simulink library "ars"  (Simulink 8.1)
settings: Solver=ode1  StartTime=0.0  StopTime=Inf  FixedStep=0.001  RelTol=1e-3
PostLoadFcn:
  | , if any(exist('dsrtsu_mdlpostloadfcn', 'file') == [2, 3, 6]), try dsrtsu_mdlpostloadfcn('Execute', bdroot); catch fprintf('Error in PostLoadFcn (dsrtsu_mdlpostloadfcn) for model "%s":\n %s\n', bdroot, lasterr); end, end,
undefined symbols (not defined in the file or in its folder): KACC_RawFMLowerLimit_mps, KACC_RawFMUpperLimit_mps
libraries: hcu_lib x2, ssc x1, ddc x1, dch x1, rsd x1, rsa x1, rst x1
settings Model: DSRTSU_INTERNAL_RTI_VER=450  DSRTSU_INTERNAL_RTI_TYPE=rti1401  RTICANMMDATA=struct('GeneralSetupData',struct('modelroot','D:\ELN150201_TAIWAN\trunk\AdasDragon\software\sw_development\arch\app\acc','generalsettings',struct('filesettings',struct('destfolder',struct('Name','RTICANMM_FILES','Check',1),'buildfolder',struct('Name','.','Check',1),'AbsDestfolder',struct('Name','D:\ELN150201_TAIWAN\trunk\AdasDragon\software\sw_development\arch\app\acc\RTICANMM_FILES'),'AbsBuildfolder',struct('Name','D:\ELN150201_TAIWAN\trunk\AdasDragon\software\sw_development\arch\app\acc'))),'options',struct('addpaths',1,'rmpaths',1,'addtrcexclusion',logical(1),'cannavigator',struct('checkmonitoring',0),'show_usrtrc',0,'use_usrtrc',0),'advanced',struct('options',[1 1 1 1 1 1 1 1 1 1 1 1 1 1 1 1 1 1 1 1 1 1 1 1 1 1 1 1 1 1 1 1 1 1 1 1 1 1 1 1 1 1 1 1 1 1 1 1 1 1 1 1 1 1 1 1 1 1 1 1 1 1 1 1 1 1 1 1 1 1 1 1 1 1 1 1 1 1 1 1 1 1 1 1 1 1 1 1 1 1 1 1 1 1 1 1 1 1 1 1]),'MPSetup',{{}},'modelname','ars','block','ars'))  DSRTSU_INTERNAL_RTIFPGA=40  Creator=tescamilla  LastModifiedBy=AT015555

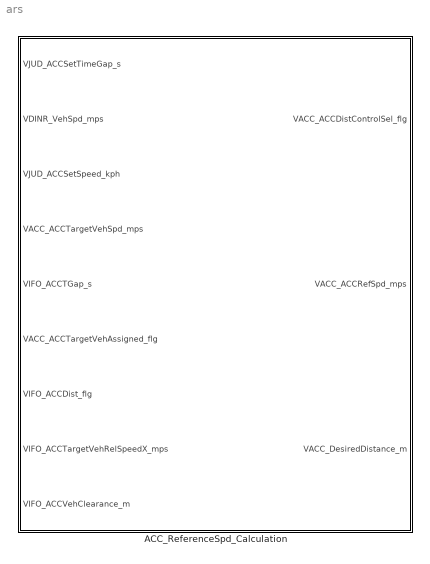
== system ars ==
  ACC_ReferenceSpd_Calculation : Subsystem

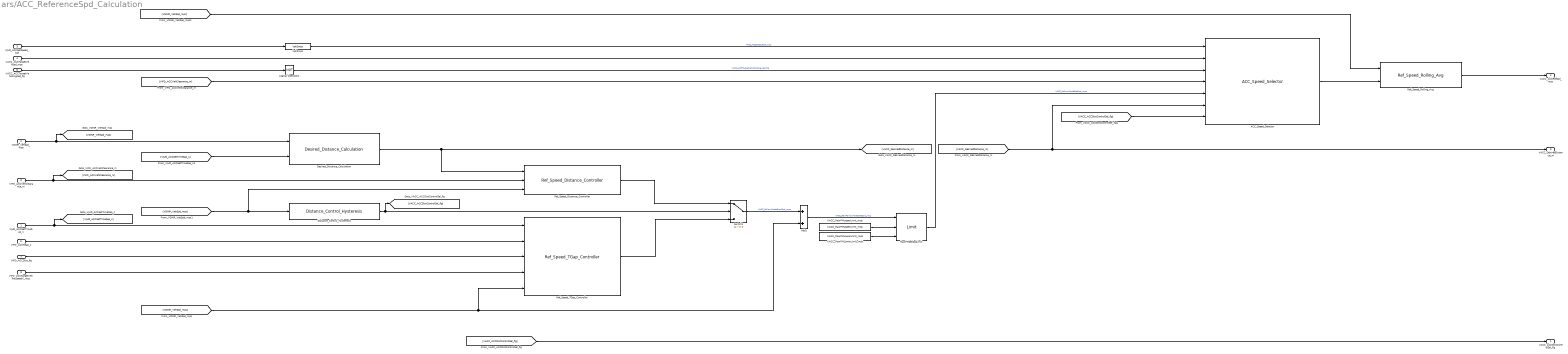
== system ars/ACC_ReferenceSpd_Calculation ==
  VJUD_ACCSetTimeGap_s : Inport
  VDINR_VehSpd_mps : Inport  Port=2
  VJUD_ACCSetSpeed_kph : Inport  Port=3
  VACC_ACCTargetVehSpd_mps : Inport  Port=4
  VIFO_ACCTGap_s : Inport  Port=5
  VACC_ACCTargetVehAssigned_flg : Inport  Port=6
  VIFO_ACCDist_flg : Inport  Port=7
  VIFO_ACCTargetVehRelSpeedX_mps : Inport  Port=8
  VIFO_ACCVehClearance_m : Inport  Port=9
  ACC_Speed_Selector : ssc/ACC_Speed_Selector
  Add1 : Sum
  Desired_Distance_Calculation : ddc/Desired_Distance_Calculation
  Distance_Control_Hysteresis : dch/Distance_Control_Hysteresis
  KACC_RawFMLowerLimit_mps : Constant  Value=KACC_RawFMLowerLimit_mps
  KACC_RawFMUpperLimit_mps : Constant  Value=KACC_RawFMUpperLimit_mps
  Logical Operator1 : Logic  Operator=NOT  AllPortsSameDT=off  OutDataTypeStr=boolean
  RawFMSetSpdLimit : hcu_lib/Limit  SystemSampleTime=-1
  Ref_Speed_Distance_Controller : rsd/Ref_Speed_Distance_Controller
  Ref_Speed_Rolling_Avg : rsa/Ref_Speed_Rolling_Avg
  Ref_Speed_TGap_Controller : rst/Ref_Speed_TGap_Controller
  Switch1 : Switch  Criteria=u2 ~= 0
  kph2mps : hcu_lib/kph2mps
  VACC_ACCDistControlSel_flg : Outport
  VACC_ACCRefSpd_mps : Outport  Port=2
  VACC_DesiredDistance_m : Outport  Port=3
  wires:
  Desired_Distance_Calculation/1 -> Ref_Speed_Distance_Controller/1, [VACC_DesiredDistance_m]
  Logical Operator1/1 -> ACC_Speed_Selector/3  "VACC_ACCTargetVehNotAssigned_flg"
  VACC_ACCTargetVehSpd_mps/1 -> ACC_Speed_Selector/2
  Ref_Speed_Rolling_Avg/1 -> VACC_ACCRefSpd_mps/1
  kph2mps/1 -> ACC_Speed_Selector/1  "VACC_ACCSetSpeed_mps"
  [VACC_DesiredDistance_m] -> VACC_DesiredDistance_m/1, ACC_Speed_Selector/6
  RawFMSetSpdLimit/1 -> ACC_Speed_Selector/5  "VACC_FollowModeSetSpd_mps"
  VJUD_ACCSetSpeed_kph/1 -> kph2mps/1
  VACC_ACCTargetVehAssigned_flg/1 -> Logical Operator1/1
  [VJUD_ACCSetTimeGap_s] -> Desired_Distance_Calculation/2
  Switch1/1 -> Add1/1  "VACC_FollowModeErrorSpd_mps"
  [VACC_ACCDistControlSel_flg] -> VACC_ACCDistControlSel_flg/1
  VIFO_ACCVehClearance_m/1 -> [VIFO_ACCVehClearance_m], Ref_Speed_Distance_Controller/2
  Ref_Speed_Distance_Controller/1 -> Switch1/1
  Ref_Speed_TGap_Controller/1 -> Switch1/3
  VJUD_ACCSetTimeGap_s/1 -> [VJUD_ACCSetTimeGap_s], Ref_Speed_TGap_Controller/1
  VIFO_ACCTGap_s/1 -> Ref_Speed_TGap_Controller/2
  VIFO_ACCDist_flg/1 -> Ref_Speed_TGap_Controller/3
  Distance_Control_Hysteresis/1 -> [VACC_ACCDistControlSel_flg], Switch1/2
  [VDINR_VehSpd_mps] -> Distance_Control_Hysteresis/1, Ref_Speed_Distance_Controller/3
  VIFO_ACCTargetVehRelSpeedX_mps/1 -> Ref_Speed_TGap_Controller/4
  Add1/1 -> RawFMSetSpdLimit/1  "VACC_RawFollowModeSetSpd_mps"
  KACC_RawFMUpperLimit_mps/1 -> RawFMSetSpdLimit/2
  KACC_RawFMLowerLimit_mps/1 -> RawFMSetSpdLimit/3
  VDINR_VehSpd_mps/1 -> [VDINR_VehSpd_mps], Desired_Distance_Calculation/1
  [VIFO_ACCVehClearance_m] -> ACC_Speed_Selector/4
  [VACC_ACCDistControlSel_flg] -> ACC_Speed_Selector/7
  ACC_Speed_Selector/1 -> Ref_Speed_Rolling_Avg/2
  [VDINR_VehSpd_mps] -> Ref_Speed_Rolling_Avg/1
  [VDINR_VehSpd_mps] -> Ref_Speed_TGap_Controller/5, Add1/2
